simulink model "TxSteering_RxMVDR_4x4_HDL_IQ"  (R2021b)
settings: Solver=FixedStepDiscrete  StartTime=0.0  StopTime=stoptime  RelTol=1e-3
PreLoadFcn:
  | model_init
InitFcn:
  | model_init
model workspace (MAT data in the model file):
  socvcb : containers.Map (value not decoded)
values from neighbouring files (symbols this model uses):
  fc = ConverterSampleRate/4    (= 491520000)    [model_init.m]
  FPGAClkRate = DataSampleRate/VectorSamplingFactor    (= 245760000)    [model_init.m]
  movavg_bitshift = nextpow2(sqrt(windowSize))    [model_init.m]
  mvdrPipelineDelay = covMatDelay+movAvgDelay+matrixDivDelay+normResponseDelay    [model_init.m]
  NCO_bits = 14    [model_init.m]
  numArrayElements = 4    [model_init.m]
  S2MM_frame_size = testSrc1.FrameLength*testSrc1.SamplesPerSymbol*3    [model_init.m]
  testSrc1 = struct()    [model_init.m]
  testSrc2 = struct()    [model_init.m]
  windowSize = 4096    [model_init.m]
undefined symbols (not defined in the file or in its folder): j, physconst
libraries: hdlsllib x19, simulink x12, dspsrcs4 x2, embsystolicmatrixops x1, embreciprocals x1, dsphdlsigops x1, commrfcorlib x1
(part 3 of 3)

== system TxSteering_RxMVDR_4x4_HDL_IQ/DUT/Rx Beamforming/MVDR/Normalize Response/MVDR Weight Update/Inner Product/Element-wise complex product ==
  u : Inport  Partition=on  PartitionDimension=1  PartitionWidth=1  PartitionOffset=0
  v : Inport  Port=2  Partition=on  PartitionDimension=1  PartitionWidth=1  PartitionOffset=0
  For Each : ForEach  DisableCoverage=on
  HDL Complex Multiply : Subsystem  mask(HDL Complex Multiplier (3 Multiply, 5 Add)){D1=2, D2=1, D3=1, D4=1, D5=1}
      mask help:
      | Xilinx devices:
      | - Set D1 = 1 or 2 to trade off speed & FF resources
      | - Set D2-D5 = 1 to fully leverage DSP48 pipelines
      | - Use sync reset
      |
      | Intel FPGAs:
      | - Set D1 = 1 or 2 depending on device family
      | - Set D5 = 1; D2, D3, D4 = 0
      | - Use async reset
      mask init:
      | delay = D1+D2+D3+D4+D5;
      mask Display:
      | fprintf('Delay=%d',delay);
      | port_label('input',1,'z1');
      | port_label('input',2,'z2');
  y : Outport  ConcatenationDimension=1
  wires:
  v/1 -> HDL Complex Multiply/2(In2)
  HDL Complex Multiply/1(Out1) -> y/1
  u/1 -> HDL Complex Multiply/1(In1)

== system TxSteering_RxMVDR_4x4_HDL_IQ/DUT/Rx Beamforming/MVDR/Normalize Response/MVDR Weight Update/Inner Product/Tree Sum with Distributed Pipelining ==
  In1 : Inport
  Delay3 : Delay  DelayLength=ceil(log2(numArrayElements))
  Tree Sum of Elements : Sum  Inputs=+  OutDataTypeStr=Inherit: Same as first input  LockScale=on
  Out1 : Outport
  wires:
  Delay3/1 -> Out1/1
  In1/1 -> Tree Sum of Elements/1
  Tree Sum of Elements/1 -> Delay3/1

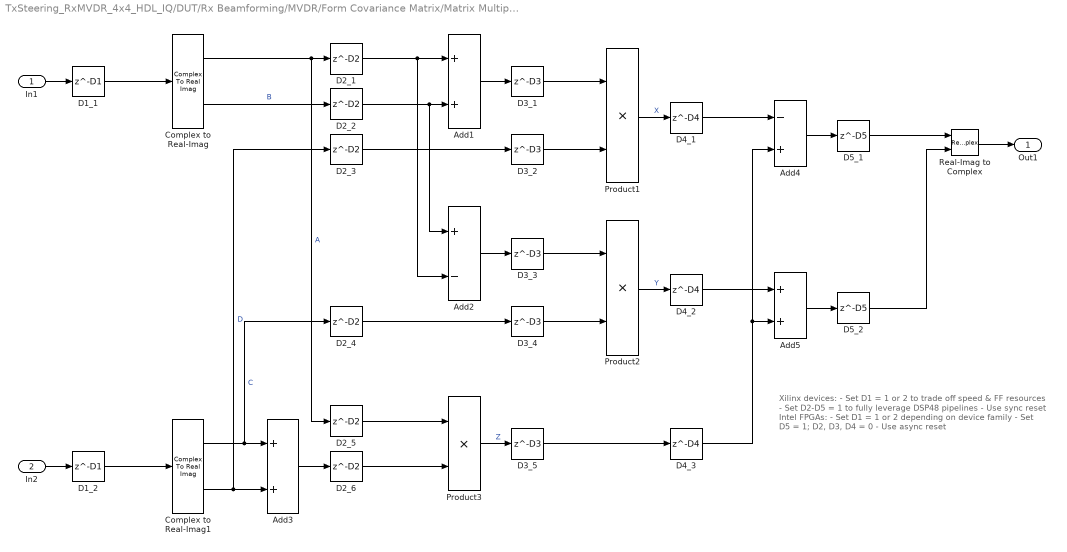
== system TxSteering_RxMVDR_4x4_HDL_IQ/DUT/Rx Beamforming/MVDR/Form Covariance Matrix/Matrix Multiply Partitioned/Partition x_conj/Partition x/HDL Complex Multiply ==
  note: Xilinx devices:
      | - Set D1 = 1 or 2 to trade off speed & FF resources
      | - Set D2-D5 = 1 to fully leverage DSP48 pipelines
      | - Use sync reset
      |
      | Intel FPGAs:
      | - Set D1 = 1 or 2 depending on device family
      | - Set D5 = 1; D2, D3, D4 = 0
      | - Use async reset
  In1 : Inport
  In2 : Inport  Port=2
  Add1 : Sum
  Add2 : Sum  Inputs=+-
  Add3 : Sum
  Add4 : Sum  Inputs=-+
  Add5 : Sum
  Complex to Real-Imag : ComplexToRealImag
  Complex to Real-Imag1 : ComplexToRealImag
  D1_1 : Delay  DelayLength=D1
  D1_2 : Delay  DelayLength=D1
  D2_{1..6} (6 alike) : Delay  DelayLength=D2
  D3_{1..5} (5 alike) : Delay  DelayLength=D3
  D4_1 : Delay  DelayLength=D4
  D4_2 : Delay  DelayLength=D4
  D4_3 : Delay  DelayLength=D4
  D5_1 : Delay  DelayLength=D5
  D5_2 : Delay  DelayLength=D5
  Product1 : Product
  Product2 : Product
  Product3 : Product
  Real-Imag to Complex : RealImagToComplex
  Out1 : Outport  VectorParamsAs1DForOutWhenUnconnected=off
  wires:
  Real-Imag to Complex/1 -> Out1/1
  In2/1 -> D1_2/1
  Complex to Real-Imag1/1 -> Add3/1, D2_4/1  "C"
  Complex to Real-Imag1/2 -> Add3/2, D2_3/1  "D"
  Product1/1 -> D4_1/1  "X"
  Product2/1 -> D4_2/1  "Y"
  Product3/1 -> D3_5/1  "Z"
  Add4/1 -> D5_1/1
  Add5/1 -> D5_2/1
  D5_1/1 -> Real-Imag to Complex/1
  D5_2/1 -> Real-Imag to Complex/2
  D4_1/1 -> Add4/1
  D4_2/1 -> Add5/1
  D3_5/1 -> D4_3/1
  Add1/1 -> D3_1/1
  Add3/1 -> D2_6/1
  Add2/1 -> D3_3/1
  Complex to Real-Imag/1 -> D2_5/1, D2_1/1  "A"
  Complex to Real-Imag/2 -> D2_2/1  "B"
  D3_1/1 -> Product1/1
  D2_6/1 -> Product3/2
  D3_3/1 -> Product2/1
  D4_3/1 -> Add4/2, Add5/2
  D3_4/1 -> Product2/2
  D3_2/1 -> Product1/2
  D2_4/1 -> D3_4/1
  D2_3/1 -> D3_2/1
  D2_5/1 -> Product3/1
  D2_2/1 -> Add1/2, Add2/1
  D2_1/1 -> Add2/2, Add1/1
  In1/1 -> D1_1/1
  D1_1/1 -> Complex to Real-Imag/1
  D1_2/1 -> Complex to Real-Imag1/1

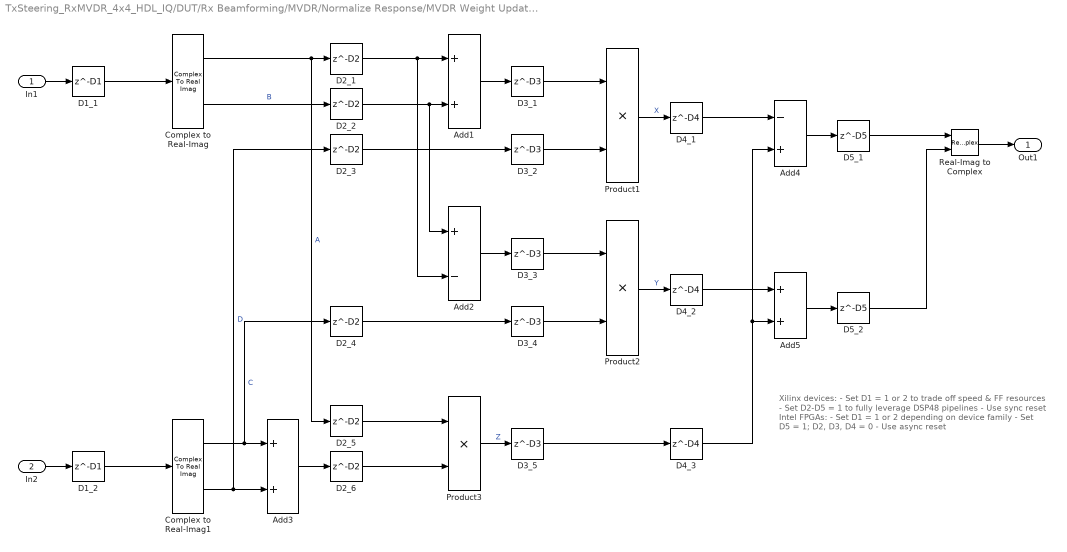
== system TxSteering_RxMVDR_4x4_HDL_IQ/DUT/Rx Beamforming/MVDR/Normalize Response/MVDR Weight Update/Inner Product/Element-wise complex product/HDL Complex Multiply ==
  note: Xilinx devices:
      | - Set D1 = 1 or 2 to trade off speed & FF resources
      | - Set D2-D5 = 1 to fully leverage DSP48 pipelines
      | - Use sync reset
      |
      | Intel FPGAs:
      | - Set D1 = 1 or 2 depending on device family
      | - Set D5 = 1; D2, D3, D4 = 0
      | - Use async reset
  In1 : Inport
  In2 : Inport  Port=2
  Add1 : Sum
  Add2 : Sum  Inputs=+-
  Add3 : Sum
  Add4 : Sum  Inputs=-+
  Add5 : Sum
  Complex to Real-Imag : ComplexToRealImag
  Complex to Real-Imag1 : ComplexToRealImag
  D1_1 : Delay  DelayLength=D1
  D1_2 : Delay  DelayLength=D1
  D2_{1..6} (6 alike) : Delay  DelayLength=D2
  D3_{1..5} (5 alike) : Delay  DelayLength=D3
  D4_1 : Delay  DelayLength=D4
  D4_2 : Delay  DelayLength=D4
  D4_3 : Delay  DelayLength=D4
  D5_1 : Delay  DelayLength=D5
  D5_2 : Delay  DelayLength=D5
  Product1 : Product  OutDataTypeStr=Inherit: Same as first input
  Product2 : Product  OutDataTypeStr=Inherit: Same as first input
  Product3 : Product  OutDataTypeStr=Inherit: Same as first input
  Real-Imag to Complex : RealImagToComplex
  Out1 : Outport  VectorParamsAs1DForOutWhenUnconnected=off
  wires:
  Real-Imag to Complex/1 -> Out1/1
  In2/1 -> D1_2/1
  Complex to Real-Imag1/1 -> Add3/1, D2_4/1  "C"
  Complex to Real-Imag1/2 -> Add3/2, D2_3/1  "D"
  Product1/1 -> D4_1/1  "X"
  Product2/1 -> D4_2/1  "Y"
  Product3/1 -> D3_5/1  "Z"
  Add4/1 -> D5_1/1
  Add5/1 -> D5_2/1
  D5_1/1 -> Real-Imag to Complex/1
  D5_2/1 -> Real-Imag to Complex/2
  D4_1/1 -> Add4/1
  D4_2/1 -> Add5/1
  D3_5/1 -> D4_3/1
  Add1/1 -> D3_1/1
  Add3/1 -> D2_6/1
  Add2/1 -> D3_3/1
  Complex to Real-Imag/1 -> D2_5/1, D2_1/1  "A"
  Complex to Real-Imag/2 -> D2_2/1  "B"
  D3_1/1 -> Product1/1
  D2_6/1 -> Product3/2
  D3_3/1 -> Product2/1
  D4_3/1 -> Add4/2, Add5/2
  D3_4/1 -> Product2/2
  D3_2/1 -> Product1/2
  D2_4/1 -> D3_4/1
  D2_3/1 -> D3_2/1
  D2_5/1 -> Product3/1
  D2_2/1 -> Add1/2, Add2/1
  D2_1/1 -> Add2/2, Add1/1
  In1/1 -> D1_1/1
  D1_1/1 -> Complex to Real-Imag/1
  D1_2/1 -> Complex to Real-Imag1/1

== matlab function TxSteering_RxMVDR_4x4_HDL_IQ/S2MM DMA Plant/AXI Stream Deserializer ==
  data: data_i input; data_o output; valid_i input; valid_o output boolean; FRAME_SIZE parameter
function [data_o, valid_o] = axis_deserializer(data_i, valid_i, FRAME_SIZE)

persistent cntr bank frame_int

if isempty(cntr)
    bank = false;
    frame_int = zeros(FRAME_SIZE, 2, 'like', data_i);
    cntr = 1;
end

% default outputs
valid_o = false;
bankidx = bank;

% Latch the frame, if we're ready to send another
if valid_i
    frame_int(cntr, bankidx+1) = data_i;
    if cntr == FRAME_SIZE
        cntr = 1;
        valid_o = true;
        bank = ~bank;
    else
        cntr = cntr + 1;
    end
end

data_o = frame_int(:,bankidx+1);

== matlab function TxSteering_RxMVDR_4x4_HDL_IQ/DUT/Rx Beamforming/MVDR/Normalize Response/MVDR Weight Update/Vector // Scalar Divide/MATLAB Function ==
  data: y input; w output; e input
function w = variableShift(y,e)
    %#codegen
    w = bitshift(y,e);
end

function C = bitshift(A,K)
%BITSHIFT Bit-wise shift.
%   C = bitshift(A, K) returns the value of fi object A
%   shifted by K bits, in fi object C.  fi object A can be any
%   fixed-point numeric type, and may either be a scalar or a
%   vector. K must be a scalar with built-in type. The
%   OverflowAction property is obeyed. The RoundingMethod is always
%   'Floor'.  
%
%   Behavior shifting off the top and bottom: If K > A.WordLength,
%   then C = upperbound(A).  If K is negative and -K >
%   A.WordLength, then C = 0.
%
%   If A is not a fi object, then C = A .* 2.^K.
    coder.inline('never')
    if isfi(A)
        if K>0
            if K>(A.WordLength-1)
                C = zeros(size(A),'like',A);
                C(:) = upperbound(A);
            else
                C = bitsll(A,K);
            end
        else
            if -K>(A.WordLength-1)
                C = zeros(size(A),'like',A);
            else
                C = bitsra(A,-K);
            end
        end
    else
        C = cast(double(A) .* 2.^double(K),'like',A);
    end
end

== matlab function TxSteering_RxMVDR_4x4_HDL_IQ/Software Interface Plant/Channel Calibration Control ==
  data: MVDRData output; MVDRValid output; dataIn input; TxNCOEnable output; validIn input; TxNCOInc output; BypassMVDR output; RxCaptureTrig output; RxCalCoeffs output; NCO_default_inc parameter
function [MVDRData,MVDRValid,TxNCOEnable,TxNCOInc,BypassMVDR,...
    RxCaptureTrig,RxCalCoeffs] = ...
    calibration_control(dataIn,validIn, NCO_default_inc)
% This state machine performs calibration on the Rx channels before
% entering into normal capture mode.

STATE_INIT = 0;
STATE_RUN_CAL = 1;
STATE_POSTCAL_DELAY = 2;
STATE_TRIG_CAPTURE = 3;
STATE_WAIT_VALID = 4;
STATE_DELAY = 5;

NUM_CHAN = 4;
FRAME_SIZE = length(dataIn)/NUM_CHAN;

persistent next_state next_count count_max
if isempty(next_state)
   next_state = STATE_INIT;
   next_count = 1;
   count_max = 100;
end

persistent TxNCOEnable_p BypassMVDR_p RxCalCoeffs_p MVDRData_p 
if isempty(TxNCOEnable_p)
    TxNCOEnable_p = true;
    BypassMVDR_p = true;
    RxCalCoeffs_p = complex(ones(NUM_CHAN, 1));
    MVDRData_p = complex(zeros(FRAME_SIZE, 1));
end

% update state variables
state = next_state;
count = next_count;

% output defaults
RxCaptureTrig = false;
MVDRValid = false;

% state transition logic
switch state
    case STATE_INIT
        if count == count_max
            next_state = STATE_RUN_CAL;
            RxCaptureTrig = true;
        else
            next_count = count + 1;
        end
    case STATE_RUN_CAL
        if validIn
            disp('Running calibration...');
            coeffs = runCal(dataIn);
            fprintf('Applying channel gains:\n');
            for ii=1:4
                fprintf('%d: scale %.2f, phase %.2f degrees\n',int32(ii),...
                    abs(coeffs(ii)),rad2deg(angle(coeffs(ii))));
            end
            RxCalCoeffs_p = coeffs;
            TxNCOEnable_p = false;
            next_state = STATE_POSTCAL_DELAY;
            next_count = 1;
            count_max = 100;
        end
    case STATE_POSTCAL_DELAY
        next_count=count+1;
        if count == count_max
            next_state = STATE_DELAY;
            BypassMVDR_p = false;
            next_count = 1;
            count_max = 4000;
        end
    case STATE_TRIG_CAPTURE
        next_state = STATE_WAIT_VALID;
        RxCaptureTrig = true;
    case STATE_WAIT_VALID
        if validIn
            next_state = STATE_DELAY;
            next_count = 1;
            count_max = 50;
            MVDRData_p = unpackMVDRData(dataIn);
            MVDRValid = true;
        end
    case STATE_DELAY
        next_count=count+1;
        if count == count_max
            next_state = STATE_TRIG_CAPTURE;
        end
end

% outputs
TxNCOInc = uint32(NCO_default_inc);
TxNCOEnable = TxNCOEnable_p;
BypassMVDR = BypassMVDR_p;
RxCalCoeffs = RxCalCoeffs_p;
MVDRData = MVDRData_p;

end


function calCoeffs = runCal(dataIn)
    % Unpack uint32 to complex int16
    temp = unpack_complex(dataIn);
    % Reshape into individual channels
    temp = reshape(temp,4,[]);
    % Make channels as columns
    temp = transpose(temp);
    % Get calibration coefficients
    calCoeffs = calibrate_channels(temp);
end

function dataOut = unpackMVDRData(dataIn)
    % reshape into individual channels
    temp = reshape(dataIn,4,[]);
    % grab real/imag from chan 1&2, discard chan 3&4
    temp = complex(temp(1,:), temp(2,:));
    % make channels as columns
    temp = transpose(temp);
    % Cast to fi and reinterpret fraction length
    temp = cast_to_fi(temp);
    temp = reinterpretcast(temp, numerictype(1,32,30));
    % Convert to double
    dataOut = double(temp);
end

== matlab function TxSteering_RxMVDR_4x4_HDL_IQ/DUT/Rx Beamforming/MVDR/Compute Weight Vector/Serialize Input Data/readyQueue ==
  data: readyEdge input; validOut output; validIn input
function validOut = readyQueue(readyEdge, validIn)

persistent readyQueued_reg
if isempty(readyQueued_reg)
    readyQueued_reg = false;
end

readyQueued = readyQueued_reg;

if readyEdge
    if validIn
        validOut = true;
    else
        validOut = false;
        readyQueued_reg = true;
    end
elseif readyQueued
    if validIn
        validOut = true;
        readyQueued_reg = false;
    else
        validOut = false; 
    end
else
    validOut = false;
end

== matlab function TxSteering_RxMVDR_4x4_HDL_IQ/DUT/Rx Beamforming/Output Selector/RepackageInput/Pack Complex Vector/pack_vector_complex ==
  data: u input; y output
function y = pack_vector_complex(u)
%#codegen

assert(~isreal(u),'Expected input to be complex');

N = coder.const(numel(u));

temp = coder.nullcopy((cast_to_fi(zeros([N*2 1],'like',real(u)))));

% Interleave real/imag
coder.unroll();
for ii=N:-1:1
    temp((ii-1)*2+2) = real(u(N-ii+1));
    temp((ii-1)*2+1) = imag(u(N-ii+1));
end

y = bitconcat(temp);

== matlab function TxSteering_RxMVDR_4x4_HDL_IQ/Software Interface Plant/Display Beamforming Patterns ==
  data: computedWeights input; signalAngle input; interfererAngle input
function updatePlot(computedWeights,signalAngle,interfererAngle)

coder.extrinsic('figure','findall','close','axes','evalin','pattern',...
    'plot_beam_patterns');

persistent hAxes sensorArray steeringVector fc

if isempty(sensorArray)
    figName = coder.const('MVDR Response Pattern');
    close(findall(0,'type','figure','name',figName));
    hFig = figure('Name',figName);
    hAxes = axes(hFig);
    sensorArray = evalin('base','sensorArray');
    steeringVector = evalin('base','steeringVector');
    fc = evalin('base','fc');
end

% Compute MVDR beamformer response
mvdrWeights = double(complex(computedWeights(1:4),computedWeights(5:8)));
mvdrResponse=pattern(sensorArray,fc,-90:90,0,'Weights',mvdrWeights);

% Compute phase shift beamformer response
phaseShiftWeights=steeringVector(fc,[signalAngle; 0]);
phaseShiftResponse=pattern(sensorArray,fc,-90:90,0,'Weights',phaseShiftWeights);

% Plot beamforming patterns
plot_beam_patterns(hAxes,mvdrResponse,phaseShiftResponse,signalAngle,interfererAngle);

== matlab function TxSteering_RxMVDR_4x4_HDL_IQ/Software Interface Plant/Process Beam Data/QPSK Receiver ==
  data: dataIn input; FrameLength parameter size=1; SamplesPerSymbol parameter size=1; PreambleLength parameter size=1; mfCoeffs parameter; rrcCoeffs parameter; dataOut output
function dataOut = qpsk_receiver(dataIn, ...
    FrameLength, SamplesPerSymbol, PreambleLength, ...
    mfCoeffs, rrcCoeffs)

dataOut = qpsk_receive(dataIn,FrameLength,SamplesPerSymbol,PreambleLength,...
    mfCoeffs, rrcCoeffs);
